simulink model "kadai22"  (R2021b)
settings: Solver=VariableStepAuto  StartTime=0.0  StopTime=1000  MaxStep=0.01  RelTol=1e-3
settings Model: Creator=is221042  LastModifiedBy=tomotomo

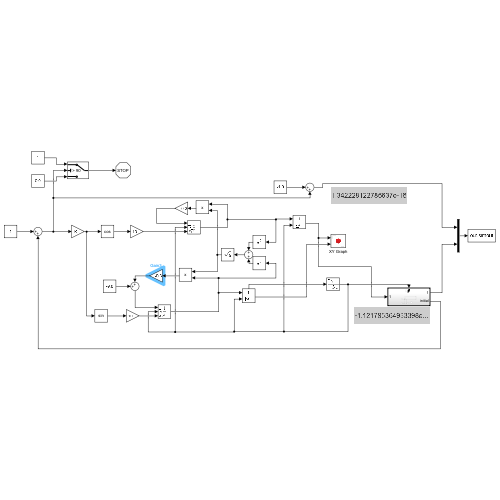
[thumbnail: Simulink's stored preview of the top-level diagram]
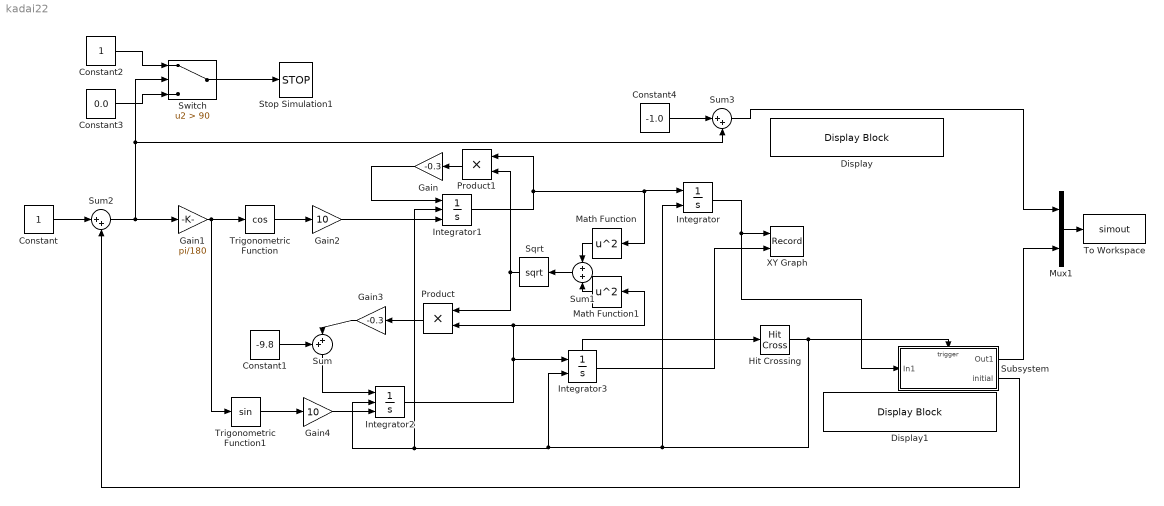
== system kadai22 ==
  Constant : Constant
  Constant1 : Constant  Value=-9.8
  Constant2 : Constant
  Constant3 : Constant  Value=0.0
  Constant4 : Constant  Value=-1.0
  Display : DisplayBlock  LabelPosition=Hide  Format=longE  Transparency=1
  Display1 : DisplayBlock  LabelPosition=Hide  Format=longE  Transparency=1
  Gain : Gain  Gain=-0.3
  Gain1 : Gain  Gain=pi/180
  Gain2 : Gain  Gain=10
  Gain3 : Gain  Gain=-0.3
  Gain4 : Gain  Gain=10
  Hit Crossing : HitCross  HitCrossingDirection=falling
  Integrator : Integrator  ExternalReset=falling
  Integrator1 : Integrator  ExternalReset=falling  InitialConditionSource=external
  Integrator2 : Integrator  ExternalReset=falling  InitialConditionSource=external
  Integrator3 : Integrator  ExternalReset=falling  ShowStatePort=on
  Math Function : Math  Operator=square  SaturateOnIntegerOverflow=on
  Math Function1 : Math  Operator=square  SaturateOnIntegerOverflow=on
  Mux1 : Mux  Inputs=2
  Product : Product
  Product1 : Product
  Sqrt : Sqrt  SaturateOnIntegerOverflow=on
  Stop Simulation1 : Stop
  Subsystem : Subsystem
  Sum : Sum  Inputs=++|
  Sum1 : Sum  Inputs=+|+
  Sum2 : Sum  Inputs=|++
  Sum3 : Sum  Inputs=|++
  Switch : Switch  Criteria=u2 > Threshold  Threshold=90
  To Workspace : ToWorkspace  VariableName=simout  SaveFormat=Timeseries  SampleTime=-1
  Trigonometric Function : Trigonometry  Operator=cos
  Trigonometric Function1 : Trigonometry
  XY Graph : Record  FileSettingsInternal="{\"entries\":[{\"content\":{\"excelSettings\":{\"content\":{},\"type\":\"Streamout.ExcelSettings\"}},\"type\":\"Streamout.FileSettingStorage\",\"uuid\":\"25803a0d-138e-4e5c-b9ed-cbfa2c072c10\"}],\"packageUris\":[\"http://schema.mathworks.com/mf0/streamout_blocks/R2020a\"],\"version\":\"1.0\"}"  Layout=[1 1]  SignalsInternal="{\"entries\":[{\"content\":{\"signals\":[{\"content\":{\"blockPath\":[\"kadai22/XY Graph\"],\"channel\":[],\"dimensions\":[1],\"domain\":\"kadai22/XY Graph\",\"lineColor\":\"#a2142f\",\"plots\":[1],\"port\":1,\"sid\":[\"\"],\"signalID\":1458,\"signalName\":\"Integrator\"},\"type\":\"RecordBlkView.Signal\",\"uuid\":\"7123b1e8-6d89-4b58-b712-76cf3f350346\"},{\"content\":{\"blockPath\":[\"kadai22/XY Graph\"],\"channel\":[],\"dimensions\":[1],\"domain\":\"kadai22/XY Graph\",\"lineColor\":\"#139fff\",\"plots\":[1],\"port\":2,\"sid\":[\"\"],\"signalID\":1462,\"signalName\":\"Integrator3:1\"},\"type\":\"RecordBlkView.Signal\",\"uuid\":\"345b0012-0e71-458e-84c5-9651380fbc3c\"}]},\"type\":\"RecordBlkView.InputSignals\",\"uuid\":\"559eb08b-8198-4c3d-a43a-dc305fecccdb\"}],\"packageUris\":[\"http://schema.mathworks.com/mf0/streamout_blocks/R2020a\"],\"version\":\"1.0\"}"  VisualizationBindings="{\"xyplotplugin\":{\"info\":[{\"series\":[{\"bindingParametersList\":[{\"parameter\":\"X-Axis\",\"signalID\":1458,\"signalName\":\"Integrator\"},{\"parameter\":\"Y-Axis\",\"signalID\":1462,\"signalName\":\"Integrator3:1\"}],\"seriesID\":57025}],\"subplotID\":1}]}}"  CompatibilityTag=XY
  wires:
  Sqrt/1 -> Product/1, Product1/2
  Integrator2/1 -> Product/2, Math Function1/1, Integrator3/1
  Math Function/1 -> Sum1/1
  Integrator3/1 -> XY Graph/2
  Product/1 -> Gain3/1
  Math Function1/1 -> Sum1/2
  Gain1/1 -> Trigonometric Function1/1, Trigonometric Function/1
  Hit Crossing/1 -> Integrator1/2, Integrator2/2, Integrator3/2, Integrator/2, Subsystem/Trigger
  Sum1/1 -> Sqrt/1
  Integrator1/1 -> Integrator/1, Math Function/1, Product1/1
  Gain2/1 -> Integrator1/3
  Gain4/1 -> Integrator2/3
  Trigonometric Function/1 -> Gain2/1
  Product1/1 -> Gain/1
  Integrator/1 -> Subsystem/1(In1), XY Graph/1
  Trigonometric Function1/1 -> Gain4/1
  Gain3/1 -> Sum/2
  Gain/1 -> Integrator1/1
  Constant1/1 -> Sum/1
  Sum/1 -> Integrator2/1
  Switch/1 -> Stop Simulation1/1
  Constant2/1 -> Switch/1
  Constant3/1 -> Switch/3
  Subsystem/1(Out1) -> Mux1/2
  Subsystem/2(initial) -> Sum2/2
  Constant4/1 -> Sum3/1
  Sum3/1 -> Mux1/1
  Constant/1 -> Sum2/1
  Sum2/1 -> Switch/2, Sum3/2, Gain1/1
  Integrator3/State -> Hit Crossing/1
  Mux1/1 -> To Workspace/1

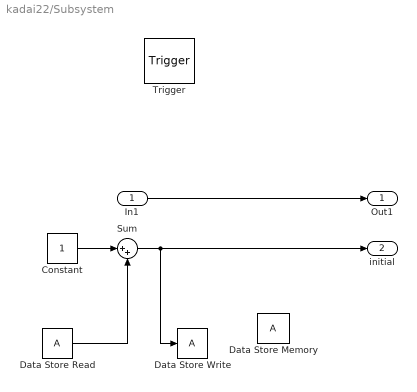
== system kadai22/Subsystem ==
  In1 : Inport
  Trigger : TriggerPort  VariantControl=(inherit)  PortDimensions=1
  Constant : Constant
  Data Store Memory : DataStoreMemory  ReadBeforeWriteMsg=warning  WriteAfterWriteMsg=warning  WriteAfterReadMsg=warning  ShowAdditionalParam=off
  Data Store Read : DataStoreRead  IndexOptions=Index vector (dialog)  Indices=1  OutputSizes=1
  Data Store Write : DataStoreWrite  IndexOptions=Index vector (dialog)  Indices=1  OutputSizes=1
  Sum : Sum  Inputs=|++
  Out1 : Outport
  initial : Outport  Port=2
  wires:
  In1/1 -> Out1/1
  Constant/1 -> Sum/1
  Sum/1 -> Data Store Write/1, initial/1
  Data Store Read/1 -> Sum/2
